simulink model "uk"  (R2013b)
settings: Solver=ode45  StartTime=0.0  StopTime=10.0  RelTol=1e-3
values from neighbouring files (symbols this model uses):
  a = 1.23999866855    [matlab.mat]    (also in qfun.m = kk(1))
  b = -4.19999658716    [matlab.mat]    (also in qfun.m = kk(2))
settings Model: Creator=labmc  LastModifiedBy=labmc

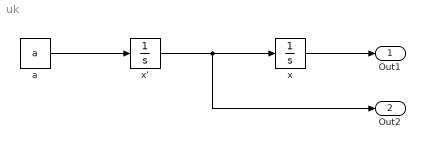
== system uk ==
  a : Constant  Value=a
  x : Integrator  InitialCondition=2
  x' : Integrator  InitialCondition=b
  Out1 : Outport
  Out2 : Outport  Port=2
  wires:
  a/1 -> x'/1
  x'/1 -> Out2/1, x/1
  x/1 -> Out1/1
